simulink model "slotineAdaptable"  (R2014b)
settings: Solver=ode45  StartTime=0.0  StopTime=15.0  MaxStep=0.1  RelTol=1e-3
undefined symbols (not defined in the file): alpha, Gamma, kd, lambda
settings Model: Creator=roberto  LastModifiedBy=roberto

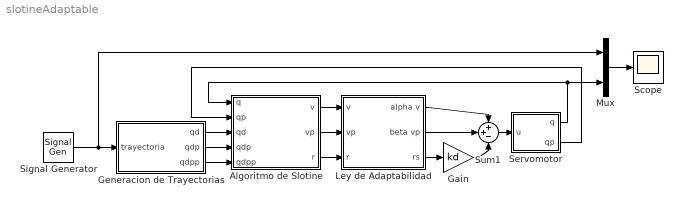
== system slotineAdaptable ==
  Algoritmo de Slotine : Subsystem
  Gain : Gain  Gain=kd
  Generacion de Trayectorias : Subsystem
  Ley de Adaptabilidad : Subsystem
  Mux : Mux  Inputs=2
  Scope : Scope
  Servomotor : Subsystem
  Signal Generator : SignalGenerator  Amplitude=0.5  Frequency=0.25
  Sum1 : Sum  Inputs=++-
  wires:
  Mux/1 -> Scope/1
  Signal Generator/1 -> Generacion de Trayectorias/1(trayectoria), Mux/1
  Generacion de Trayectorias/1(qd) -> Algoritmo de Slotine/3(qd)
  Generacion de Trayectorias/2(qdp) -> Algoritmo de Slotine/4(qdp)
  Generacion de Trayectorias/3(qdpp) -> Algoritmo de Slotine/5(qdpp)
  Sum1/1 -> Servomotor/1(u)
  Servomotor/1(q) -> Mux/2, Algoritmo de Slotine/1(q)
  Servomotor/2(qp) -> Algoritmo de Slotine/2(qp)
  Algoritmo de Slotine/1(v) -> Ley de Adaptabilidad/1(v)
  Algoritmo de Slotine/2(vp) -> Ley de Adaptabilidad/2(vp)
  Algoritmo de Slotine/3(r) -> Ley de Adaptabilidad/3(r)
  Ley de Adaptabilidad/2(beta vp) -> Sum1/2
  Ley de Adaptabilidad/1(alpha v) -> Sum1/1
  Ley de Adaptabilidad/3(rs) -> Gain/1
  Gain/1 -> Sum1/3

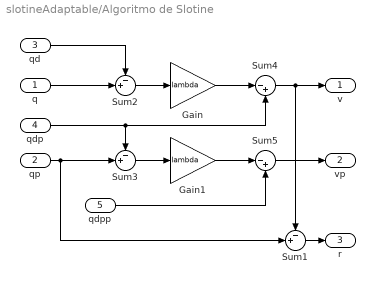
== system slotineAdaptable/Algoritmo de Slotine ==
  q : Inport
  qp : Inport  Port=2
  qd : Inport  Port=3
  qdp : Inport  Port=4
  qdpp : Inport  Port=5
  Gain : Gain  Gain=lambda
  Gain1 : Gain  Gain=lambda
  Sum1 : Sum  Inputs=-+|
  Sum2 : Sum  Inputs=-+|
  Sum3 : Sum  Inputs=-+|
  Sum4 : Sum  Inputs=|-+
  Sum5 : Sum  Inputs=|-+
  v : Outport
  vp : Outport  Port=2
  r : Outport  Port=3
  wires:
  Gain/1 -> Sum4/1
  qp/1 -> Sum1/2, Sum3/2
  Sum4/1 -> Sum1/1, v/1
  q/1 -> Sum2/2
  Sum5/1 -> vp/1
  Sum3/1 -> Gain1/1
  Gain1/1 -> Sum5/1
  Sum2/1 -> Gain/1
  qdpp/1 -> Sum5/2
  qdp/1 -> Sum3/1, Sum4/2
  qd/1 -> Sum2/1
  Sum1/1 -> r/1

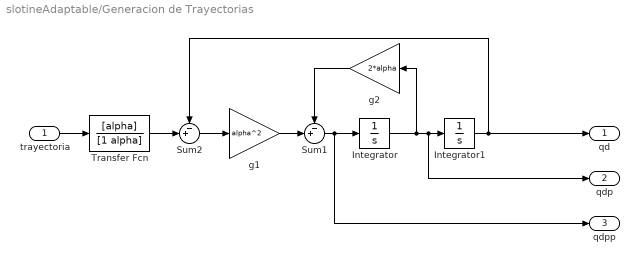
== system slotineAdaptable/Generacion de Trayectorias ==
  trayectoria : Inport
  Integrator : Integrator
  Integrator1 : Integrator
  Sum1 : Sum  Inputs=-+|
  Sum2 : Sum  Inputs=-+|
  Transfer Fcn : TransferFcn  Numerator=[alpha]  Denominator=[1 alpha]
  g1 : Gain  Gain=alpha^2
  g2 : Gain  Gain=2*alpha
  qd : Outport
  qdp : Outport  Port=2
  qdpp : Outport  Port=3
  wires:
  Sum2/1 -> g1/1
  trayectoria/1 -> Transfer Fcn/1
  Integrator1/1 -> qd/1, Sum2/1
  Integrator/1 -> g2/1, qdp/1, Integrator1/1
  g1/1 -> Sum1/2
  Sum1/1 -> qdpp/1, Integrator/1
  g2/1 -> Sum1/1
  Transfer Fcn/1 -> Sum2/2

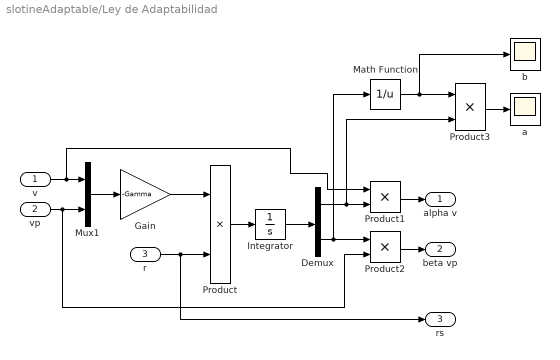
== system slotineAdaptable/Ley de Adaptabilidad ==
  v : Inport
  vp : Inport  Port=2
  r : Inport  Port=3
  Demux : Demux  Outputs=2
  Gain : Gain  Gain=-Gamma
  Integrator : Integrator
  Math Function : Math  Operator=reciprocal  SaturateOnIntegerOverflow=on
  Mux1 : Mux  Inputs=2
  Product{,1..3} (4 alike) : Product
  a : Scope
      settings: TimeRange=15  YMin=-0.004195011337868496  YMax=0.35
  b : Scope
      settings: TimeRange=15  YMin=0  YMax=54.08814334444835  SaveName=ScopeData2
  alpha v : Outport
  beta vp : Outport  Port=2
  rs : Outport  Port=3
  wires:
  Gain/1 -> Product/1
  r/1 -> rs/1, Product/2
  vp/1 -> Product2/2, Mux1/2
  Mux1/1 -> Gain/1
  v/1 -> Product1/1, Mux1/1
  Product1/1 -> alpha v/1
  Product2/1 -> beta vp/1
  Demux/2 -> Math Function/1, Product2/1
  Demux/1 -> Product3/2, Product1/2
  Math Function/1 -> b/1, Product3/1
  Product3/1 -> a/1
  Product/1 -> Integrator/1
  Integrator/1 -> Demux/1

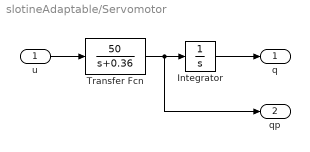
== system slotineAdaptable/Servomotor ==
  u : Inport
  Integrator : Integrator
  Transfer Fcn : TransferFcn  Numerator=[50]  Denominator=[1 0.36]
  q : Outport
  qp : Outport  Port=2
  wires:
  Transfer Fcn/1 -> Integrator/1, qp/1
  u/1 -> Transfer Fcn/1
  Integrator/1 -> q/1
